simulink model "third"  (R2024a)
settings: Solver=VariableStepAuto  StartTime=0.0  StopTime=10  RelTol=1e-3
values from neighbouring files (symbols this model uses):
  A = 5    [third_calc.m]
  Am = [0 1 0; 0 0 1; 1 -3 3]    [third_calc.m]
  B = 5.5    [third_calc.m]
  C = 1.5    [third_calc.m]
  ksi = [ksi10; ksi20; ksi30]    [third_calc.m]
  T = 0.2    [first_calc.m]    (also in second.m; third_calc.m = 0.25)
settings Model: Creator=ventus  LastModifiedBy=ventus

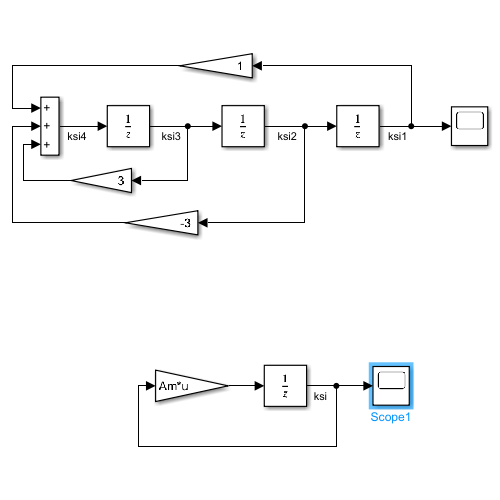
[thumbnail: Simulink's stored preview of the top-level diagram]
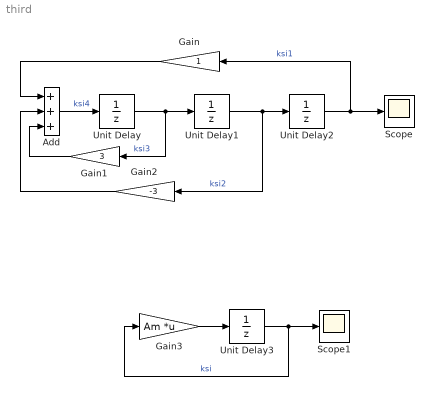
== system third ==
  Add : Sum  Inputs=+++
  Gain : Gain
  Gain1 : Gain  Gain=3
  Gain2 : Gain  Gain=-3
  Gain3 : Gain  Gain=Am  Multiplication=Matrix(K*u)
  Scope : Scope
  Scope1 : Scope
  Unit Delay : UnitDelay  InitialCondition=A + 2*B*T + 3*C*T^2  SampleTime=T  HasFrameUpgradeWarning=on
  Unit Delay1 : UnitDelay  InitialCondition=A + B*T + C*T^2  SampleTime=T  HasFrameUpgradeWarning=on
  Unit Delay2 : UnitDelay  InitialCondition=A  SampleTime=T  HasFrameUpgradeWarning=on
  Unit Delay3 : UnitDelay  InitialCondition=ksi  SampleTime=T  HasFrameUpgradeWarning=on
  wires:
  Unit Delay/1 -> Unit Delay1/1, Gain1/1  "ksi3"
  Unit Delay1/1 -> Unit Delay2/1, Gain2/1  "ksi2"
  Unit Delay2/1 -> Scope/1, Gain/1  "ksi1"
  Add/1 -> Unit Delay/1  "ksi4"
  Gain/1 -> Add/1
  Gain1/1 -> Add/3
  Gain2/1 -> Add/2
  Gain3/1 -> Unit Delay3/1
  Unit Delay3/1 -> Scope1/1, Gain3/1  "ksi"
